simulink model "simu71"  (R2018a)
settings: Solver=VariableStepAuto  StartTime=0.0  StopTime=10.0  RelTol=1e-3
values from neighbouring files (symbols this model uses):
  omega = 4    [TimeResponseof1stn2ndorder.m]    (also in pgo7.m)
  zeta = 2    [TimeResponseof1stn2ndorder.m]    (also in TimeResponseof2ndordersystem.m = 1.2; pg08.m = 1.2; pgo7.m)
libraries: simulink x1
settings Model: Creator=SHRUTI  LastModifiedBy=SHRUTI

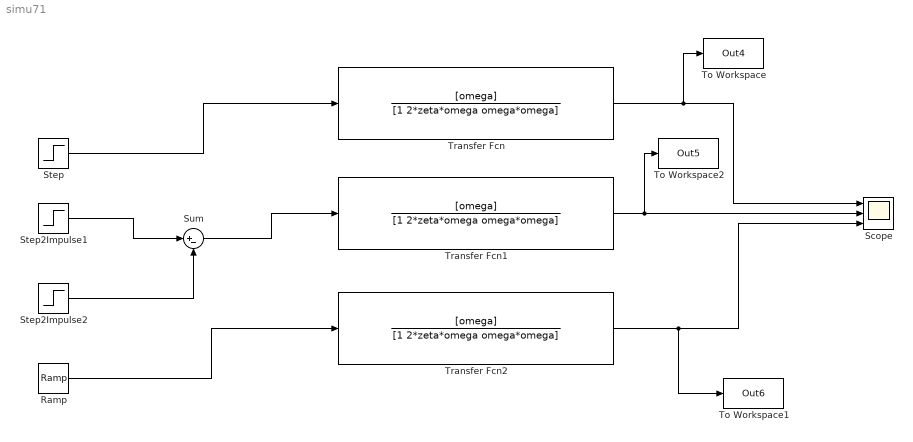
== system simu71 ==
  Ramp : simulink/Sources/Ramp  slope=1  start=0  InitialOutput=0
  Scope : Scope  NumInputPorts=3
  Step : Step  SampleTime=0
  "Step2Impulse1 " : Step  SampleTime=0
  Step2Impulse2 : Step  SampleTime=0
  Sum : Sum  Inputs=|+-
  To Workspace : ToWorkspace  VariableName=Out4  SampleTime=-1
  To Workspace1 : ToWorkspace  VariableName=Out6  SampleTime=-1
  To Workspace2 : ToWorkspace  VariableName=Out5  SampleTime=-1
  Transfer Fcn : TransferFcn  Numerator=[omega]  Denominator=[1 2*zeta*omega omega*omega]
  Transfer Fcn1 : TransferFcn  Numerator=[omega]  Denominator=[1 2*zeta*omega omega*omega]
  Transfer Fcn2 : TransferFcn  Numerator=[omega]  Denominator=[1 2*zeta*omega omega*omega]
  wires:
  "Step2Impulse1 "/1 -> Sum/1
  Step2Impulse2/1 -> Sum/2
  Sum/1 -> Transfer Fcn1/1
  Step/1 -> Transfer Fcn/1
  Transfer Fcn/1 -> To Workspace/1, Scope/1
  Transfer Fcn1/1 -> Scope/2, To Workspace2/1
  Transfer Fcn2/1 -> To Workspace1/1, Scope/3
  Ramp/1 -> Transfer Fcn2/1
